simulink model "SingularityAvoidance"  (R2022a)
settings: Solver=ode4  StartTime=0.0  StopTime=Inf  FixedStep=1/500  RelTol=1e-3
InitFcn:
  | home = [0.45; 0; 0.49];
  | 
  | A = [ 0; 0.45; 0.3];
  | B = [ 0; -0.45; 0.3];
  | 
  | %A = [ 0.1; 0.6; 0.3];
  | %B = [ -0.1; -0.6; 0.3];
  | 
  | %A = [ 0.55; 0.1; 0.3];
  | %B = [ -0.1; -0.55; 0.3];
  | 
  | %A = [ -0.1; 0.6; 0.3];
  | %B = [ -0.1; -0.6; 0.3];
  | 
  | T = 20;
undefined symbols (not defined in the file): DiscIntNeverNeededParam, HIL, qc_get_step_size
libraries: quarc_library x5, simulink x2
settings Model: ExtModeTrigDuration=10000  Creator=fvranes  LastModifiedBy=lgonzalez
settings SolverCC: AlgebraicLoopSolver=TrustRegion
settings DataIOCC: ReturnWorkspaceOutputs=off
settings DebuggingCC: UnderspecifiedInitializationDetection=Classic  MergeDetectMultiDrivingBlocksExec=none  UnconnectedInputMsg=warning  UnconnectedOutputMsg=warning  UnconnectedLineMsg=warning
settings ModelReferenceCC: PropagateSignalLabelsOutOfModel=off
settings SFSimCC: CustomCodeUndefinedFunction=UseInterfaceOnly

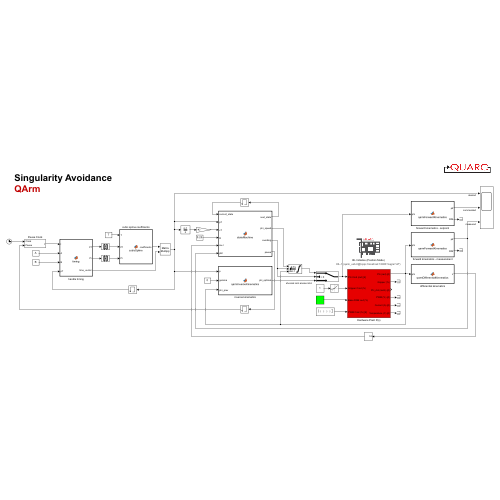
[thumbnail: Simulink's stored preview of the top-level diagram]
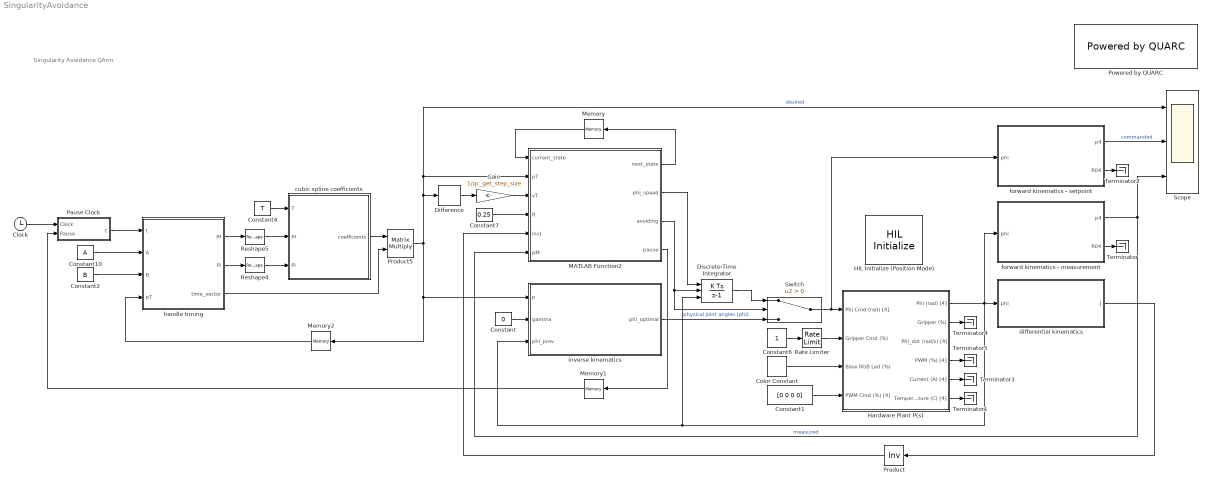
== system SingularityAvoidance ==
  note: Singularity Avoidance
      | QArm
  Clock : Clock
  Color Constant : quarc_library/Sources/Signals/Color Constant  color=[0 1 0]
      settings: SourceProductName=QUARC Targets
  Constant : Constant  Value=0
  Constant1 : Constant  Value=[0 0 0 0]
  Constant10 : Constant  Value=A  VectorParams1D=off
  Constant2 : Constant  Value=B  VectorParams1D=off
  Constant4 : Constant  Value=T  VectorParams1D=off
  Constant6 : Constant
  Constant7 : Constant  Value=0.25
  Difference : simulink/Discrete/Difference  ICPrevInput=0.0  OutMin=[]  OutMax=[]  OutDataType=fixdt(1, 16)  OutScaling=2^-10  DoSatur=off
  Discrete-Time Integrator : DiscreteIntegrator  ExternalReset=rising  InitialConditionSource=external  SampleTime=-1  LimitOutput=on  UpperSaturationLimit=[170 85 85 180]*pi/180  LowerSaturationLimit=[-170 -85 -95 -180]*pi/180  ICPrevOutput=DiscIntNeverNeededParam  ICPrevScaledInput=DiscIntNeverNeededParam
  Gain : Gain  Gain=1/qc_get_step_size
  HIL Initialize (Position Mode) : quarc_library/Data Acquisition/Generic/Configuration/HIL Initialize  object_name=HIL-1  board_type=qarm_usb  board_number=0@tcpip://localhost:18900?nagle='off'  board_options=j0_mode=0;j1_mode=0;j2_mode=0;j3_mode=0;gripper_mode=0;  exclusive=off  active=on  hardware_clocks=[0]  clock_modes=[]  initial_clock_frequencies=[]  set_clock_params_at_start=off  set_clock_params_at_switch_in=off  set_clock_frequencies_at_start=off  set_clock_frequencies_at_switch_in=off  analog_input_channels=[5:9]  analog_input_configurations=[]  analog_input_maximums=[]  analog_input_minimums=[]  set_analog_input_params_at_start=off  set_analog_input_params_at_switch_in=off  analog_output_channels=[]  analog_output_maximums=inf  analog_output_minimums=-inf  initial_analog_outputs=[0]  final_analog_outputs=[0]  watchdog_analog_outputs=[]  set_analog_output_params_at_start=off  set_analog_output_params_at_switch_in=off  set_analog_outputs_at_start=off  set_analog_outputs_at_switch_in=off  set_analog_outputs_at_terminate=off  set_analog_outputs_at_switch_out=off  set_analog_outputs_on_watchdog=off  digital_input_channels=[]  digital_output_channels=[]  digital_output_configuration=[]  initial_digital_outputs=[0]  final_digital_outputs=[0]  watchdog_digital_outputs=[0]  set_digital_output_params_at_start=off  set_digital_output_params_at_switch_in=off  set_digital_outputs_at_start=off  set_digital_outputs_at_switch_in=off  set_digital_outputs_at_terminate=off  set_digital_outputs_at_switch_out=off  set_digital_outputs_on_watchdog=off  encoder_channels=[]  quadrature=[]  encoder_filter_frequency=[]  initial_encoder_counts=[]  set_encoder_params_at_start=off  set_encoder_params_at_switch_in=off  set_encoder_counts_at_start=off  set_encoder_counts_at_switch_in=off  pwm_channels=[]  pwm_modes=[]  pwm_frequency=[]  pwm_configuration=[]  pwm_alignment=[]  pwm_polarity=[]  pwm_leading_deadband=[]  pwm_trailing_deadband=[]  initial_pwm_outputs=[]  final_pwm_outputs=[]  watchdog_pwm_outputs=[]  set_pwm_params_at_start=off  set_pwm_params_at_switch_in=off  set_pwm_outputs_at_start=off  set_pwm_outputs_at_switch_in=off  set_pwm_outputs_at_terminate=off  set_pwm_outputs_at_switch_out=off  set_pwm_outputs_on_watchdog=off  other_output_channels=[1000:1004 11000:11003 11005:11007]  initial_other_outputs=[zeros(1,9), ones(1,3)]  final_other_outputs=[zeros(1,9), ones(1,3)]  watchdog_other_outputs=zeros(1,12)  set_other_outputs_at_start=off  set_other_outputs_at_switch_in=off  set_other_outputs_at_terminate=on  set_other_outputs_at_switch_out=off  set_other_outputs_on_watchdog=off
  Hardware Plant P(s) : Subsystem
  MATLAB Function2 : MATLAB Function  TreatAsAtomicUnit=on
  Memory : Memory  InitialCondition=1
  Memory1 : Memory  InitialCondition=1
  Memory2 : Memory  InitialCondition=1
  Pause Clock : Subsystem
  Powered by QUARC : quarc_library/Logos/Powered by QUARC
  Product : Product  Inputs=/  Multiplication=Matrix(*)
  Product5 : Product  Multiplication=Matrix(*)
  Rate Limiter : RateLimiter  SampleTimeMode=inherited
  Reshape4 : Reshape  OutputDimensionality=Column vector (2-D)
  Reshape5 : Reshape  OutputDimensionality=Column vector (2-D)
  Scope : Scope  NumInputPorts=3
  Switch : Switch  Criteria=u2 > Threshold  SaturateOnIntegerOverflow=off  InputSameDT=off
  Terminator{,1..5} (6 alike) : Terminator
  cubic spline coefficients : MATLAB Function  TreatAsAtomicUnit=on
  differential kinematics : MATLAB Function  TreatAsAtomicUnit=on
  forward kinematics - measurement : MATLAB Function  TreatAsAtomicUnit=on
  forward kinematics - setpoint : MATLAB Function  TreatAsAtomicUnit=on
  handle timing : MATLAB Function  TreatAsAtomicUnit=on
  inverse kinematics : MATLAB Function  TreatAsAtomicUnit=on
  wires:
  Hardware Plant P(s)/4(PWM (%) [4]) -> Terminator5/1
  Hardware Plant P(s)/6(Temperature (C) [4]) -> Terminator1/1
  inverse kinematics/1(phi_optimal) -> Switch/3  "physical joint angles (phi)"
  Rate Limiter/1 -> Hardware Plant P(s)/2(Gripper Cmd (%))
  Hardware Plant P(s)/5(Current (A) [4]) -> Terminator3/1
  Color Constant/1 -> Hardware Plant P(s)/3(Base RGB Led (%))
  Constant1/1 -> Hardware Plant P(s)/4(PWM Cmd (%) [4])
  Constant6/1 -> Rate Limiter/1
  Hardware Plant P(s)/2(Gripper (%)) -> Terminator4/1
  Constant/1 -> inverse kinematics/2(gamma)
  forward kinematics - measurement/1(p4) -> Scope/3, MATLAB Function2/6(pM)  "measured"
  differential kinematics/1(J) -> Product/1
  Product/1 -> MATLAB Function2/5(invJ)
  Reshape4/1 -> cubic spline coefficients/3(Pi)
  Clock/1 -> Pause Clock/1(Clock)
  cubic spline coefficients/1(coefficients) -> Product5/1
  Constant4/1 -> cubic spline coefficients/1(T)
  handle timing/3(time_vector) -> Product5/2
  Reshape5/1 -> cubic spline coefficients/2(Pf)
  Constant7/1 -> MATLAB Function2/4(R)
  Switch/1 -> forward kinematics - setpoint/1(phi), Hardware Plant P(s)/1(Phi Cmd (rad) [4])
  Product5/1 -> inverse kinematics/1(p), Memory2/1, Scope/1, MATLAB Function2/2(pT), Difference/1  "desired"
  MATLAB Function2/3(avoiding) -> Discrete-Time Integrator/2, Switch/2
  Discrete-Time Integrator/1 -> Switch/1
  MATLAB Function2/2(phi_speed) -> Discrete-Time Integrator/1
  Hardware Plant P(s)/1(Phi (rad) [4]) -> differential kinematics/1(phi), Discrete-Time Integrator/3, inverse kinematics/3(phi_prev), forward kinematics - measurement/1(phi)
  forward kinematics - measurement/2(R04) -> Terminator/1
  Difference/1 -> Gain/1
  Gain/1 -> MATLAB Function2/3(vT)
  forward kinematics - setpoint/2(R04) -> Terminator2/1
  Memory/1 -> MATLAB Function2/1(current_state)
  MATLAB Function2/1(next_state) -> Memory/1
  forward kinematics - setpoint/1(p4) -> Scope/2  "commanded"
  Pause Clock/1(t) -> handle timing/1(t)
  MATLAB Function2/4(pause) -> Memory1/1
  Memory1/1 -> Pause Clock/2(Pause)
  handle timing/2(Pi) -> Reshape4/1
  handle timing/1(Pf) -> Reshape5/1
  Constant10/1 -> handle timing/2(A)
  Constant2/1 -> handle timing/3(B)
  Memory2/1 -> handle timing/4(pT)

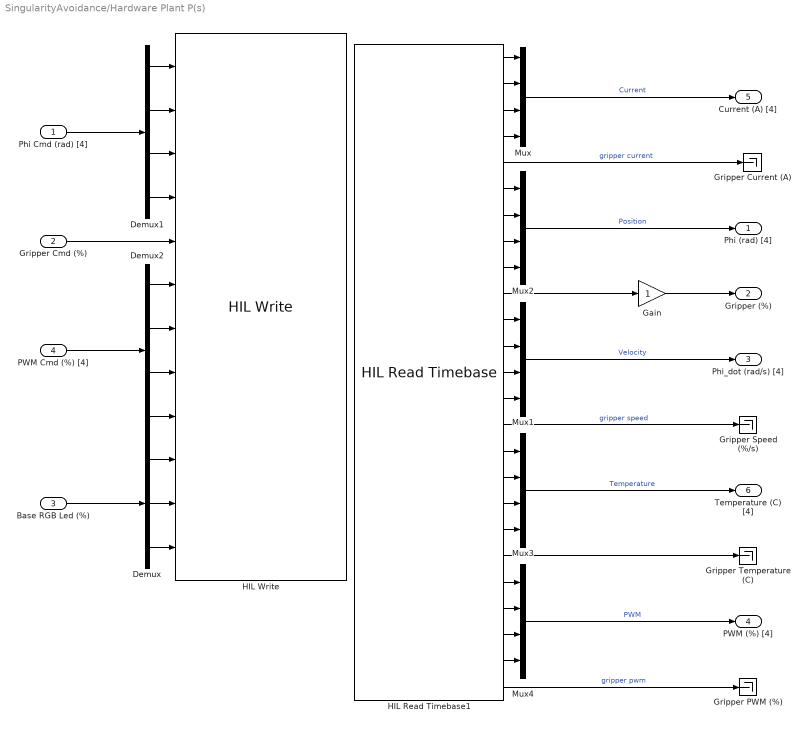
== system SingularityAvoidance/Hardware Plant P(s) ==
  Phi Cmd (rad) [4] : Inport
  Gripper Cmd (%) : Inport  Port=2
  Base RGB Led (%) : Inport  Port=3
  PWM Cmd (%) [4] : Inport  Port=4
  Demux : Demux  Outputs=3
  Demux1 : Demux
  Demux2 : Demux
  Gain : Gain
  Gripper Current (A) : Terminator
  Gripper PWM (%) : Terminator
  Gripper Speed (%/s) : Terminator
  Gripper Temperature (C) : Terminator
  HIL Read Timebase1 : quarc_library/Data Acquisition/Generic/Timebases/HIL Read Timebase  object_name=HIL-1  clock=0  analog_channels=[5:9]  encoder_channels=[]  digital_channels=[]  other_channels=[1000:1004 3000:3004 10000:10004 11000:11004]  active=on  vector_output=off  data_type_mode=Inherit via back propagation  encoder_data_type=double  digital_data_type=boolean  overflow_mode=Synchronize (for simulated cards only)  samples_in_buffer=1
  HIL Write : quarc_library/Data Acquisition/Generic/Immediate I//O/HIL Write  object_name=HIL-1  analog_channels=[]  pwm_channels=[]  digital_channels=[]  other_channels=[1000:1004 11000:11003 11005:11007]  sample_time=-1  active=on  vector_input=off
  Mux{,1..4} (5 alike) : Mux
  Phi (rad) [4] : Outport  VectorParamsAs1DForOutWhenUnconnected=off
  Gripper (%) : Outport  Port=2  VectorParamsAs1DForOutWhenUnconnected=off
  Phi_dot (rad/s) [4] : Outport  Port=3  VectorParamsAs1DForOutWhenUnconnected=off
  PWM (%) [4] : Outport  Port=4  VectorParamsAs1DForOutWhenUnconnected=off
  Current (A) [4] : Outport  Port=5  VectorParamsAs1DForOutWhenUnconnected=off
  Temperature (C) [4] : Outport  Port=6  VectorParamsAs1DForOutWhenUnconnected=off
  wires:
  HIL Read Timebase1/14 -> Mux1/4
  HIL Read Timebase1/9 -> Mux2/4
  HIL Read Timebase1/6 -> Mux2/1
  HIL Read Timebase1/18 -> Mux3/3
  HIL Read Timebase1/8 -> Mux2/3
  HIL Read Timebase1/12 -> Mux1/2
  HIL Read Timebase1/4 -> Mux/4
  HIL Read Timebase1/7 -> Mux2/2
  HIL Read Timebase1/5 -> Gripper Current (A)/1  "gripper current"
  HIL Read Timebase1/15 -> Gripper Speed (%/s)/1  "gripper speed"
  Demux/3 -> HIL Write/12
  HIL Read Timebase1/3 -> Mux/3
  HIL Read Timebase1/17 -> Mux3/2
  HIL Read Timebase1/16 -> Mux3/1
  HIL Read Timebase1/11 -> Mux1/1
  Demux/1 -> HIL Write/10
  HIL Read Timebase1/19 -> Mux3/4
  Demux/2 -> HIL Write/11
  HIL Read Timebase1/13 -> Mux1/3
  HIL Read Timebase1/2 -> Mux/2
  HIL Read Timebase1/1 -> Mux/1
  HIL Read Timebase1/20 -> Gripper Temperature (C)/1
  Mux/1 -> Current (A) [4]/1  "Current"
  Mux1/1 -> Phi_dot (rad/s) [4]/1  "Velocity"
  Mux3/1 -> Temperature (C) [4]/1  "Temperature"
  Base RGB Led (%)/1 -> Demux/1
  Demux1/1 -> HIL Write/1
  Demux1/2 -> HIL Write/2
  Demux1/3 -> HIL Write/3
  Demux1/4 -> HIL Write/4
  Phi Cmd (rad) [4]/1 -> Demux1/1
  PWM Cmd (%) [4]/1 -> Demux2/1
  Demux2/1 -> HIL Write/6
  Demux2/2 -> HIL Write/7
  Demux2/3 -> HIL Write/8
  Demux2/4 -> HIL Write/9
  Mux2/1 -> Phi (rad) [4]/1  "Position"
  HIL Read Timebase1/21 -> Mux4/1
  HIL Read Timebase1/22 -> Mux4/2
  HIL Read Timebase1/23 -> Mux4/3
  HIL Read Timebase1/24 -> Mux4/4
  HIL Read Timebase1/25 -> Gripper PWM (%)/1  "gripper pwm"
  Mux4/1 -> PWM (%) [4]/1  "PWM"
  HIL Read Timebase1/10 -> Gain/1
  Gain/1 -> Gripper (%)/1
  Gripper Cmd (%)/1 -> HIL Write/5

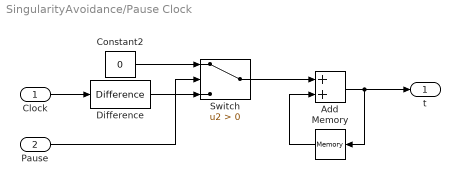
== system SingularityAvoidance/Pause Clock ==
  Clock : Inport
  Pause : Inport  Port=2
  Add : Sum
  Constant2 : Constant  Value=0
  Difference : simulink/Discrete/Difference  ICPrevInput=0.0  OutMin=[]  OutMax=[]  OutDataType=fixdt(1, 16)  OutScaling=2^-10  DoSatur=off
  Memory : Memory
  Switch : Switch  Criteria=u2 > Threshold  SaturateOnIntegerOverflow=off  InputSameDT=off
  t : Outport  VectorParamsAs1DForOutWhenUnconnected=off
  wires:
  Clock/1 -> Difference/1
  Add/1 -> t/1, Memory/1
  Difference/1 -> Switch/3
  Memory/1 -> Add/2
  Pause/1 -> Switch/2
  Switch/1 -> Add/1
  Constant2/1 -> Switch/1

== matlab function SingularityAvoidance/differential kinematics ==
  data: phi input; J output
function J   = qarmDifferentialKinematics(phi)

%% QUANSER_ARM_FDK
% v 1.0 - 13th August 2020

% REFERENCE: 
% Chapter 5. Velocity Kinematics
% Robot Dynamics and Control 
% Spong, Vidyasagar
% 1989

% INPUTS:
% phi     : Alternate joint angles vector 4 x 1

% OUTPUTS:
% p4      : End-effector frame {4} position vector expressed in base frame {0}
% R04     : rotation matrix from end-effector frame {4} to base frame {0}

%% Manipulator parameters:
L1 = 0.1400;
L2 = 0.3500;
L3 = 0.0500;
L4 = 0.2500;
L5 = 0.1500;

%% Alternate parameters
l1 = L1;
l2 = sqrt(L2^2 + L3^2);
l3 = L4 + L5;
beta = atan(L3/L2);

%% From phi space to theta space 
theta = phi;
theta(1) = phi(1);
theta(2) = phi(2) + beta - pi/2;
theta(3) = phi(3) - beta;
theta(4) = phi(4);

%% Jacobian term definition:

J = eye(4);
J(1,1) = ; 
J(1,2) = ; 
J(1,3) = ; 
J(1,4) = ;
J(2,1) = ; 
J(2,2) = ;
J(2,3) = ;
J(2,4) = ;
J(3,1) = ;
J(3,2) = ;
J(3,3) = ;
J(3,4) = ;
J(4,1) = ;
J(4,2) = ;
J(4,3) = ;
J(4,4) = ;

end

== matlab function SingularityAvoidance/cubic spline coefficients ==
  data: T input; coefficients output; Pf input; Pi input
function coefficients = cubicSpline(T, Pf, Pi)

% Cubic spline coefficients for X, Y and Z (coloumns)
a0 = [ ; ; ];
a1 = [ ; ; ];
a2 = [ ; ; ];
a3 = [ ; ; ];

% Output coefficients as a 3 x 4 matrix (1 row each for x, y and z)
coefficients = [a0, a1, a2, a3];

== matlab function SingularityAvoidance/forward kinematics - measurement ==
  data: phi input; p4 output; R04 output
function [p4, R04] = qarmForwardKinematics(phi)

%% QUANSER_ARM_FPK
% v 4.0 - 4th June 2020

% REFERENCE: 
% Chapter 3. Forward Kinematics
% Robot Dynamics and Control 
% Spong, Vidyasagar
% 1989

% INPUTS:
% phi     : Alternate joint angles vector 4 x 1

% OUTPUTS:
% p4      : End-effector frame {4} position vector expressed in base frame {0}
% R04     : rotation matrix from end-effector frame {4} to base frame {0}

%% Manipulator parameters:
L1 = 0.1400;
L2 = 0.3500;
L3 = 0.0500;
L4 = 0.2500;
L5 = 0.1500;

%% Alternate parameters
l1 = ;
l2 = ;
l3 = ;
beta = ;

%% From phi space to theta space 
theta = phi;
theta(1) = phi(1);
theta(2) = phi(2);
theta(3) = phi(3);
theta(4) = phi(4);

%% Transformation matrices for all frames:

% T{i-1}{i} = quanser_arm_DH(  a, alpha,  d,     theta );
        T01 = quanser_arm_DH(  0,     0,  0,         0 );
        T12 = quanser_arm_DH(  0,     0,  0,         0 );
        T23 = quanser_arm_DH(  0,     0,  0,         0 );
        T34 = quanser_arm_DH(  0,     0,  0,         0 );

        T02 = ;
        T03 = ;
        T04 = ;

%% Position of end-effector Transformation

% Extract the Position vector 
p4 = ;

% Extract the Rotation matrix
R04 = ;

end

function T = quanser_arm_DH(a,alpha,d,theta)

%% QUANSER_ARM_DH
% v 1.0 - 26th March 2019

% REFERENCE: 
% Chapter 3. Forward and Inverse Kinematics
% Robot Modeling and Control 
% Spong, Hutchinson, Vidyasagar
% 2006

% INPUTS:
% a       :   translation  : along : x_{i}   : from : z_{i-1} : to : z_{i}
% alpha   :      rotation  : about : x_{i}   : from : z_{i-1} : to : z_{i}
% d       :   translation  : along : z_{i-1} : from : x_{i-1} : to : x_{i}
% theta   :      rotation  : about : z_{i-1} : from : x_{i-1} : to : x_{i}
% NOTE: Standard DH Parameters

% OUTPUTS:
% T       : transformation                   : from :     {i} : to : {i-1}

%%
% Rotation Transformation about z axis by theta
T_R_z = ;
     
% Translation Transformation along z axis by d
T_T_z = ;

% Translation Transformation along x axis by a
T_T_x = ;

% Rotation Transformation about x axis by alpha
T_R_x = ;

% For a transformation FROM frame {i} TO frame {i-1}: A
% rotate about z, 
% then translate along z, 
% then translate along x, 
% lastly, rotate about x
T = ;

end

== matlab function SingularityAvoidance/inverse kinematics ==
  data: p input; gamma input; phi_optimal output; phi_prev input
function phi_optimal   = qarmInverseKinematics(p, gamma, phi_prev)

%% QUANSER_ARM_IPK
% v 4.0 - 4th June 2020

% REFERENCE: 
% Chapter 4. Inverse Kinematics
% Robot Dynamics and Control 
% Spong, Vidyasagar
% 1989

% INPUTS:
% p        : end-effector position vector expressed in base frame {0}
% gamma    : wrist rotation angle gamma

% OUTPUTS:
% phi_optimal : Best solution depending on phi_prev
% phi         : All four Inverse Kinematics solutions as a 4x4 matrix. 
%               Each col is a solution.

%% Manipulator parameters:
L1 = 0.1400;
L2 = 0.3500;
L3 = 0.0500;
L4 = 0.2500;
L5 = 0.1500;
beta = ;

%% Alternate parameters
lambda1 = ;
lambda2 = ;
lambda3 = ;

%% Initialization
theta = zeros(4, 4);
phi = zeros(4, 4);

%% Joint angle 2 and 3: 
% Equations:
    % lambda2 cos(theta2) + (-lambda3) sin(theta2 + theta3) = sqrt(x^2 + y^2)
    %   A     cos( 2    ) +     C      sin(   2   +    3  ) =    D
    
    % lambda2 sin(theta2) - (-lambda3) cos(theta2 + theta3) = lambda1 - z
    %   A     sin( 2    ) -     C      cos(   2   +    3  ) =    H

% Solution:
    A = ;
    C = ;
    H = ;
    D1 = ;
    D2 = ;
    F = ;

    theta(3,1) = 2*atan2( C + sqrt(C^2 - F^2) , F );
	theta(3,2) = 2*atan2( C - sqrt(C^2 - F^2) , F );
    theta(3,3) = theta(3,1);
	theta(3,4) = theta(3,2);

    M = ;
    N = ;
    cos_term = ;
    sin_term = ;
    theta(2,1) = atan2(sin_term, cos_term);

    M = ;
    N = ;
    cos_term = ;
    sin_term = ;
    theta(2,2) = atan2(sin_term, cos_term);

    M = ;
    N = ;
    cos_term = ;
    sin_term = ;
    theta(2,3) = atan2(sin_term, cos_term);

    M = ;
    N = ;
    cos_term = ;
    sin_term = ;
    theta(2,4) = atan2(sin_term, cos_term);


%% Joint angle 1:
% Equation:
    % y / x = tan(theta1);

% Solution
    theta(1,1) = ;
    theta(1,2) = ;
    theta(1,3) = ;
    theta(1,4) = ;
    
%% Remap theta back to phi
phi(1,:) = ;
phi(2,:) = ;
phi(3,:) = ;
phi(4,:) = ;

phi = mod(phi + pi, 2*pi) - pi;

phi_optimal = phi(:,1);
if norm(phi_optimal - phi_prev) > norm(phi(:,2) - phi_prev)
    phi_optimal = phi(:,2);
end
if norm(phi_optimal - phi_prev) > norm(phi(:,3) - phi_prev)
    phi_optimal = phi(:,3);
end
if norm(phi_optimal - phi_prev) > norm(phi(:,4) - phi_prev)
    phi_optimal = phi(:,4);
end

end

== matlab function SingularityAvoidance/handle timing ==
  data: Pf output size=[3,1]; Pi output size=[3,1]; t input; time_vector output; A input; B input; pT input
function [Pf, Pi, time_vector] = timing(t, A, B, pT)

Pf = zeros(3,1);
Pi = zeros(3,1);
persistent time_bias
persistent final
persistent initial
persistent temp

if isempty(final)
    final = B; 
    initial = [0.45;0;0.49];
    temp = A;
    time_bias = 0;
end

% Swap final and initial positions when the target gets to final
if norm(pT - final, 2) < 0.001
    % Handle first case for home separately
    if norm(initial -[0.45;0;0.49], 2) == 0
        initial = A;
    end

    % Swap initial and final positions
    temp = final;
    final = initial;
    initial = temp;
    time_bias = t;
end

Pf = final;
Pi = initial;

% Keep the timer constrained
t = t - time_bias;

% time vector 
time_vector = [1;t;t^2;t^3];

== matlab function SingularityAvoidance/forward kinematics - setpoint ==
  data: phi input; p4 output; R04 output
function [p4, R04] = qarmForwardKinematics(phi)

%% QUANSER_ARM_FPK
% v 4.0 - 4th June 2020

% REFERENCE: 
% Chapter 3. Forward Kinematics
% Robot Dynamics and Control 
% Spong, Vidyasagar
% 1989

% INPUTS:
% phi     : Alternate joint angles vector 4 x 1

% OUTPUTS:
% p4      : End-effector frame {4} position vector expressed in base frame {0}
% R04     : rotation matrix from end-effector frame {4} to base frame {0}

%% Manipulator parameters:
L1 = 0.1400;
L2 = 0.3500;
L3 = 0.0500;
L4 = 0.2500;
L5 = 0.1500;

%% Alternate parameters
l1 = ;
l2 = ;
l3 = ;
beta = ;

%% From phi space to theta space 
theta = phi;
theta(1) = phi(1);
theta(2) = phi(2);
theta(3) = phi(3);
theta(4) = phi(4);

%% Transformation matrices for all frames:

% T{i-1}{i} = quanser_arm_DH(  a, alpha,  d,     theta );
        T01 = quanser_arm_DH(  0,     0,  0,         0 );
        T12 = quanser_arm_DH(  0,     0,  0,         0 );
        T23 = quanser_arm_DH(  0,     0,  0,         0 );
        T34 = quanser_arm_DH(  0,     0,  0,         0 );

        T02 = ;
        T03 = ;
        T04 = ;

%% Position of end-effector Transformation

% Extract the Position vector 
p4 = ;

% Extract the Rotation matrix
R04 = ;

end

function T = quanser_arm_DH(a,alpha,d,theta)

%% QUANSER_ARM_DH
% v 1.0 - 26th March 2019

% REFERENCE: 
% Chapter 3. Forward and Inverse Kinematics
% Robot Modeling and Control 
% Spong, Hutchinson, Vidyasagar
% 2006

% INPUTS:
% a       :   translation  : along : x_{i}   : from : z_{i-1} : to : z_{i}
% alpha   :      rotation  : about : x_{i}   : from : z_{i-1} : to : z_{i}
% d       :   translation  : along : z_{i-1} : from : x_{i-1} : to : x_{i}
% theta   :      rotation  : about : z_{i-1} : from : x_{i-1} : to : x_{i}
% NOTE: Standard DH Parameters

% OUTPUTS:
% T       : transformation                   : from :     {i} : to : {i-1}

%%
% Rotation Transformation about z axis by theta
T_R_z = ;
     
% Translation Transformation along z axis by d
T_T_z = ;

% Translation Transformation along x axis by a
T_T_x = ;

% Rotation Transformation about x axis by alpha
T_R_x = ;

% For a transformation FROM frame {i} TO frame {i-1}: A
% rotate about z, 
% then translate along z, 
% then translate along x, 
% lastly, rotate about x
T = ;

end

== matlab function SingularityAvoidance/MATLAB Function2 ==
  settings: updateMethod=DISCRETE
  data: next_state output; phi_speed output; avoiding output size=1; current_state input; pT input; vT input; R input; invJ input; pM input; pause output
function [next_state, phi_speed, avoiding, pause] = stateMachine(current_state, pT, vT, R, invJ, pM)

persistent rate output
if isempty(rate)
    rate = 0;
    output = [0;0;0];
end
pause = 0;
insideCircle = norm(pT(1:2),2) <= R;

switch current_state
    
    % Outside Avoidance Zone
    case 1 
        % State Transition
        if insideCircle
            next_state = ;
        else
            next_state = ;
        end
        
        % State Action
        phi_speed = ;
        avoiding = ;
    
	% Move to target
    case 2 
        % State Computation Logic
        allRoots = roots([vT(1)^2+vT(2)^2, 2*(vT(1)*pT(1)+vT(2)*pT(2)), pT(1)^2 + pT(2)^2 - R^2]);
        solutions = real(allRoots);
        idx = 1;
        if solutions(2) >= solutions(1)
            idx = 2;
        end
        maxTime = max(solutions(idx), 0.002);
        output = [pT(1:2,1) + vT(1:2,1)*maxTime; pT(3)];
        maxAngle = atan2(output(2), output(1)) - atan2(pT(2), pT(1));          
        rate = maxAngle/maxTime;

        % State Transition
        next_state = ;
        
        % State Action
        phi_speed = ;
        avoiding = ;
    
	% Wait at target
    case 3 
        % State Computation Logic (if target is close to output, wait for
        % arm to get close first befor proceeding)
%         if norm(pT - output, 2) < 0.001
%             pause = 1;
%         end
        
        % State Transition
        if norm(pM - output, 2) < 0.01
            next_state = 4;
        else
            next_state = 3;            
        end
        
        % State Action
        phi_speed = ;
        avoiding = ;
	
	% Exit Strategy
    case 4 
        % State Transition
        if norm(pT(1:2), 2) > R
            next_state = ;
        else
            next_state = ;
        end
        
        % State Action
        phi_speed = ;
        avoiding = ;
	
	% Default Case
    otherwise
        % State Transition
        next_state = current_state;    
        
        % State Action
        phi_speed = [0; 0; 0; 0];
        avoiding = 0;
        
end
